simulink model "compass"  (R2016a)
settings: Solver=FixedStepAuto  StartTime=0.0  StopTime=inf  RelTol=1e-3
settings Model: SimulationMode=external  Creator=IceDragon  LastModifiedBy=hanan
settings SolverCC: PositivePriorityOrder=on
settings OptimizationCC: OptimizeModelRefInitCode=on  LifeSpan=1  MaxStackSize=64
settings HardwareCC: ProdBitPerPointer=32  ProdLargestAtomicInteger=Long  ProdLargestAtomicFloat=Double  ProdWordSize=32  ProdHWDeviceType=ARM Compatible->ARM Cortex
settings RTWCC: SystemTargetFile=ert.tlc  HardwareBoard=Raspberry Pi  TemplateMakefile=ert_default_tmf  CustomInclude=bridge simucopter  CustomSource=simucopter-agent.cpp BridgeClient.cpp ZmqBridgeMessageSerializer.cpp AbstractBridgeCommandHandler.cpp BridgeMessage.cpp  CustomDefine=SIMULINK_AGENT  CustomInitializer=simucopter_init();  CustomTerminator=simucopter_stop();  Toolchain=GNU GCC Raspberry Pi  BuildConfiguration=Specify  TargetLang=C++
settings CodeAppCC: ForceParamTrailComments=on  OperatorAnnotations=on  SimulinkDataObjDesc=on  SFDataObjDesc=on  MATLABFcnDesc=on  MangleLength=10  InsertBlockDesc=on  MATLABSourceComments=on
settings ERTTargetCC: SupportVariableSizeSignals=on  ExtModeMexArgs='10.66.66.254' 0 17725  RootIOFormat=Structure reference  IndentSize=4

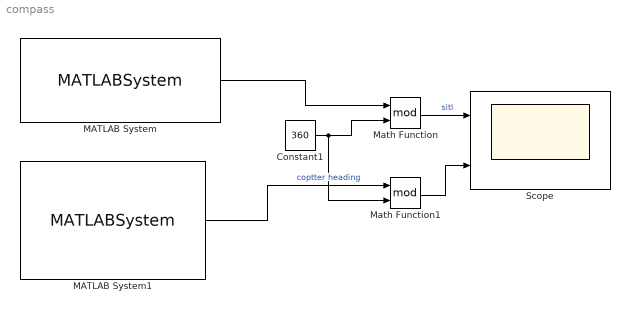
== system compass ==
  Constant1 : Constant  Value=360
  MATLAB System : MATLABSystem  System=sitl_heading  SimulateUsing=Code generation
      mask Type: sitl_heading
      mask Display:
      | disp('sitl_heading');
      | port_label('output',1,'degrees');
  MATLAB System1 : MATLABSystem  System=copter_heading  SimulateUsing=Code generation
      mask Type: copter_heading
      mask Display:
      | disp('copter_heading');
      | port_label('output',1,'degrees');
  Math Function : Math  Operator=mod  SaturateOnIntegerOverflow=on
  Math Function1 : Math  Operator=mod  SaturateOnIntegerOverflow=on
  Scope : Scope  NumInputPorts=2
  wires:
  MATLAB System/1 -> Math Function/1
  Math Function/1 -> Scope/1  "sitl"
  Constant1/1 -> Math Function1/2, Math Function/2
  MATLAB System1/1 -> Math Function1/1  "coptter heading"
  Math Function1/1 -> Scope/2
